simulink model "Lab1_2"  (R2021a)
settings: Solver=ode45  StartTime=0.0  StopTime=10000/20e6  RelTol=1e-3  EnableMultiTasking=on
undefined symbols (not defined in the file): fdesignblkfcn, gcbh, xlfda_numerator
libraries: hdlBasic x3, xbsIndex_r4 x1, dsparch4 x1, hdlUtilities x1
settings Model: Creator=danielm  LastModifiedBy=kv25
settings SolverCC: AlgebraicLoopSolver=TrustRegion
settings DataIOCC: LimitDataPoints=on  SaveFormat=Array  ReturnWorkspaceOutputs=off
settings OptimizationCC: LifeSpan=inf
settings DebuggingCC: UnderspecifiedInitializationDetection=Classic  MergeDetectMultiDrivingBlocksExec=none  SolverPrmCheckMsg=warning  AllowSymbolicDim=off  SFUnexpectedBacktrackingDiag=warning  SFNoUnconditionalDefaultTransitionDiag=warning  SFExecutionAtInitializationDiag=none  SFMachineParentedDataDiag=warning  ArithmeticOperatorsInVariantConditions=warning
settings HardwareCC: ProdBitPerPointer=32  ProdBitPerSizeT=32  ProdBitPerPtrDiffT=32  ProdLargestAtomicFloat=None  ProdIntDivRoundTo=Undefined  ProdEndianess=Unspecified  ProdWordSize=32  ProdHWDeviceType=32-bit Generic
settings ModelReferenceCC: PropagateSignalLabelsOutOfModel=off
settings SFSimCC: SimUseLocalCustomCode=off  CustomCodeUndefinedFunction=UseInterfaceOnly
settings RTWCC: RTWUseLocalCustomCode=off
settings CodeAppCC: StateflowObjectComments=on
settings GRTTargetCC: TargetLangStandard=C89/C90 (ANSI)
settings ConfigComp: CovMetricSettings=dw  CovSaveCumulativeToWorkspaceVar=on  CovSaveSingleToWorkspaceVar=on  CovExternalEMLEnable=off  CovSFcnEnable=off

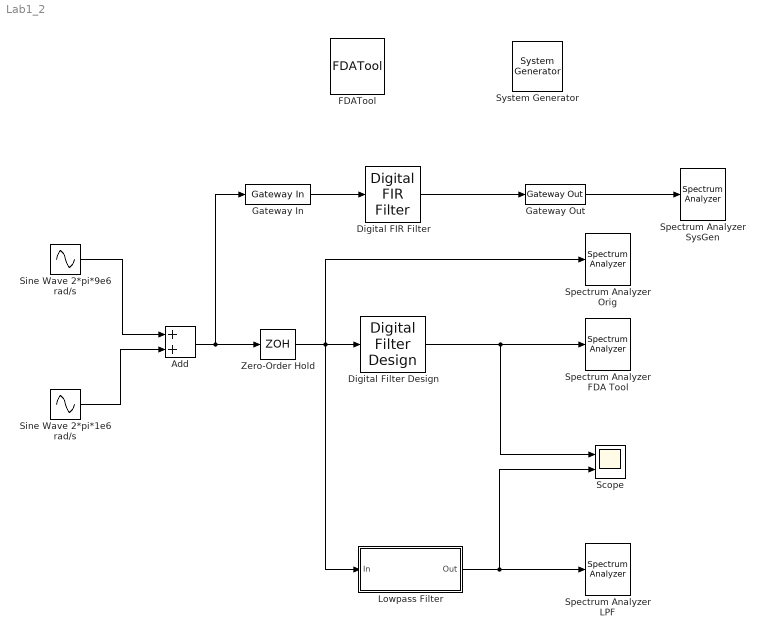
== system Lab1_2 ==
  " System Generator" : xbsIndex_r4/ System Generator  Tag=genX  xilinxfamily=zynq  part=xc7z020  speed=-1  package=clg484  synthesis_tool=Vivado  clock_wrapper=Clock Enables  directory=./netlist  proj_type=Vivado  Synth_file=Vivado Synthesis Defaults  Impl_file=Vivado Implementation Defaults  testbench=off  simulink_period=1/120e6  sysclk_period=8.33  dcm_input_clock_period=10  incr_netlist=off  trim_vbits=Everywhere in SubSystem  dbl_ovrd=According to Block Masks  core_generation=According to Block Masks  run_coregen=off  deprecated_control=off  eval_field=0  block_type=sysgen
  Add : Sum
  Digital Filter Design : dsparch4/Digital Filter Design  mwdsp_browser_bugfix_var=off
  Digital FIR Filter : hdlBasic/Digital FIR Filter  coeff_source=off  coefficientvector=xlfda_numerator('FDATool')  coeff_calulate=on  coefficient_width=19  coefficient_fractional_bits=19  interpolation_filter_rate=1  decimation_filter_rate=1  fda_coefficientvector=[-0.0024 -0.0042 0.0095 0.0200 -0.0380 -0.0696 0.1374 0.4472 0.4472 0.1374 -0.0696 -0.0380 0.0200 0.0095 -0.0042 -0.0024]  simulation_type=fast_sim  simulation_model=sysgen:fir_macro  XmcBlockStatus=1  maskContainerNames=group1  block_type=fir_macro  block_config=sysgen:fir_macro_config
  FDATool : hdlUtilities/FDATool  block_type=fdatool
      settings: infoedit=FDATool
  Gateway In : hdlBasic/Gateway In  gui_display_data_type=Fixed-point  arith_type=Signed (2's comp)  n_bits=num_bits  bin_pt=bin_pt  preci_type=Single  exp_width=8  frac_width=24  rows=1  columns=1  quantization="Round  (unbiased: +/- Inf)"  overflow=Saturate  period=1/20e6  UseAsADC=off  ADCChannel='1'  interface=None  automatic_assignment=on  address_offset=hex2dec('00')  intf_name=''  intf_description=''  default_value=0  timing_constraint=None  locs_specified=off  LOCs={}  io_standard={}  inherit_from_input=off  hdl_port=on  XmcBlockStatus=1  maskContainerNames=group4  block_type=gatewayin  block_config=sysgen:gateway_in_config  block_width_w=590  block_height_w=620  block_width=640  block_height=850
  Gateway Out : hdlBasic/Gateway Out  inherit_from_input=off  hdl_port=on  rows=1  columns=1  UseAsDAC=off  DACChannel='1'  interface=None  automatic_assignment=on  address_offset=hex2dec('00')  intf_name=''  intf_description=''  timing_constraint=None  locs_specified=off  LOCs={}  io_standard={}  XmcBlockStatus=1  maskContainerNames=group4  block_type=gatewayout  block_config=sysgen:gateway_out_config  block_width_w=590  block_height_w=620  block_width=620  block_height=750
  Lowpass Filter : Subsystem  DialogController=fdesignblkfcn  InitFcn=fdesignblkfcn(gcbh, {'InitFcn'});  mask(Lowpass Filter){}
      mask help: Design a lowpass filter
      settings: CopyFcn=fdesignblkfcn(gcbh, {'CopyFcn'});
      mask Help: helpview(mapfilelocation('dsp'), 'dsplowpassfilter');
      mask Display: disp('Lowpass')
  Scope : Scope  NumInputPorts=2
  Sine Wave 2*pi*1e6 rad/s : Sin  Frequency=2*pi*1e6  SampleTime=0
  Sine Wave 2*pi*9e6 rad/s : Sin  Frequency=2*pi*9e6  SampleTime=0
  Spectrum Analyzer FDA Tool : SpectrumAnalyzer
  Spectrum Analyzer LPF : SpectrumAnalyzer
  Spectrum Analyzer Orig : SpectrumAnalyzer
  "Spectrum Analyzer SysGen " : SpectrumAnalyzer
  Zero-Order Hold : ZeroOrderHold  SampleTime=1/20e6
  wires:
  Sine Wave 2*pi*9e6 rad/s/1 -> Add/1
  Sine Wave 2*pi*1e6 rad/s/1 -> Add/2
  Digital Filter Design/1 -> Scope/1, Spectrum Analyzer FDA Tool/1
  Zero-Order Hold/1 -> Spectrum Analyzer Orig/1, Lowpass Filter/1(In), Digital Filter Design/1
  Lowpass Filter/1(Out) -> Scope/2, Spectrum Analyzer LPF/1
  Add/1 -> Gateway In/1, Zero-Order Hold/1
  Gateway In/1 -> Digital FIR Filter/1
  Digital FIR Filter/1 -> Gateway Out/1
  Gateway Out/1 -> "Spectrum Analyzer SysGen "/1

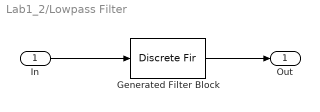
== system Lab1_2/Lowpass Filter ==
  In : Inport
  Generated Filter Block : DiscreteFir  Tag=BlockMethodSubSystem  Coefficients=[0.006802019168867246 -0.0018271019166862348 -0.051845131678638426 0.0057350837125695478 0.29497742250115677 0.49199741364352395 0.29497742250115677 0.0057350837125695478 -0.051845131678638426 -0.0018271019166862348 0.006802019168867246]  InputProcessing=Columns as channels (frame based)
  Out : Outport  VectorParamsAs1DForOutWhenUnconnected=off
  wires:
  In/1 -> Generated Filter Block/1
  Generated Filter Block/1 -> Out/1
